simulink model "SPGF_FSK_0000_R2020b"  (R2020b)
settings: Solver=ode4  StartTime=0.0  StopTime=1.4  FixedStep=50e-6/50  RelTol=1e-3  EnableMultiTasking=on
undefined symbols (not defined in the file): D11, Delta
libraries: powerlib x2546, powerlib_meascontrol x183, simulink x24
(part 5 of 34)

== system SPGF_FSK_0000_R2020b/W15 ==
  DPL : Subsystem  Commented=on  mask{N=6, Frequency=[50], R_matrix=[0.615576503610254 0.0494305423965082 0.0494304372287521 0.0494304372287521 0.0494304372287521 0.0494304372287521;0.0494305423965082 0.673800204514058 0.0494304372287521 0.0494304372287521 0.0494304372287521 0.0494304372287521;0.0494304372287521 0.0494304372287521 0.615577059271979 0.0494310980582332 0.0494309929448645 0.0494309929448645;0.0494304372287521 0.0494304372287521 0.0494310980582332 0.673800760175783 0.0494309929448645 0.0494309929448645;0.0494304372287521 0.0494304372287521 0.0494309929448645 0.0494309929448645 0.615577059271979 0.0494310980582332;0.0494304372287521 0.0494304372287521 0.0494309929448645 0.0494309929448645 0.0494310980582332 0.673800760175783], L_matrix=[0.00267974020684065 0.00245992521794015 0.00224611545694793 0.00224611545694793 0.00224611545694793 0.00224611545694793;0.00245992521794015 0.00245824456959281 0.00224611545694793 0.00224611545694793 0.00224611545694793 0.00224611545694793;0.00224611545694793 0.00224611545694793 0.00260525290490007 0.00238543791599956 0.00226842802338409 0.00226842802338409;0.00224611545694793 0.00224611545694793 0.00238543791599956 0.00238375726765222 0.00226842802338409 0.00226842802338409;0.00224611545694793 0.00224611545694793 0.00226842802338409 0.00226842802338409 0.00260525290490007 0.00238543791599956;0.00224611545694793 0.00224611545694793 0.00226842802338409 0.00226842802338409 0.00238543791599956 0.00238375726765222], C_matrix=[1.52007862009692e-07 -1.52007862009692e-07 0 0 0 0;-1.52007862009692e-07 3.21528164058002e-07 0 0 0 0;0 0 1.52007862009692e-07 -1.52007862009692e-07 0 0;0 0 -1.52007862009692e-07 3.21528164058002e-07 0 0;0 0 0 0 1.52007862009692e-07 -1.52007862009692e-07;0 0 0 0 -1.52007862009692e-07 3.21528164058002e-07], Rg_matrix=[1047017.83833883 -1047017.83833883 Inf Inf Inf -Inf;-1047017.83833883 494995.340635804 Inf Inf Inf -Inf;Inf Inf 1047017.83833883 -1047017.83833883 Inf -Inf;Inf Inf -1047017.83833883 494995.340635804 Inf -Inf;Inf Inf Inf Inf 1047017.83833883 -1047017.83833883;Inf Inf Inf Inf -1047017.83833883 494995.340635804], LineLength=[0.5]}
      mask prompts: N "Number of phases [N]"; Frequency "Frequency used for rlc specification [Hz]:"; R_matrix "Resistance per unit length [Ohms/km] NxN matrix"; L_matrix "Inductance per unit length [H/km] NxN matrix"; C_matrix "Capacitance per unit length [F/km] NxN matrix"; Rg_matrix "Resistance shunt matrix 6*6 [Ohm*km]"; LineLength "Line Length(km)"
      mask init:
      | % Rloss=1/(2*pi*Frequency*C_matrix(1,1)*TangLoss);
      | Rg_matrix=Rg_matrix./LineLength;
      mask Display:
      | port_label('lconn',1,'A');
      | port_label('lconn',2,'B');
      | port_label('lconn',3,'C');
      | 
      | port_label('rconn',1,'a');
      | port_label('rconn',2,'b');
      | port_label('rconn',3,'c');
      | 
      | disp('1x50');
  Pi : Subsystem  mask{R0=0.589, X0=0.09, Cp0=0.29, tg=2, Frequency=[50], LineLength=[0.5]}
      mask prompts: R0 "Удельное активное сопротивление, Ом/км"; X0 "Удельное индуктивное сопротивление, Ом/км"; Cp0 "Удельная рабочая емкость, мкФ/км"; tg "Тангенс диэлектрических потерь, %"; Frequency "Частота сети, Гц"; LineLength "Длина линии, км"
      mask init:
      | R=R0*LineLength;
      | L=X0*LineLength/(2*pi*Frequency);
      | Cp=Cp0*LineLength*1e-6;
      | Cmf=0.1525*Cp;
      | Cfg=0.56*Cp;
      | tg_pu=tg/100;
      | 
      | Rmf=1/(Cmf*2*pi*Frequency*tg_pu);
      | Rfg=1/(Cfg*2*pi*Frequency*tg_pu);
      mask Display:
      | port_label('lconn',1,'A');
      | port_label('lconn',2,'B');
      | port_label('lconn',3,'C');
      | 
      | port_label('rconn',1,'a');
      | port_label('rconn',2,'b');
      | port_label('rconn',3,'c');
      | 
      | disp('1x50');
  Q : Subsystem
  concentrated : Subsystem  Commented=on  mask{N=6, Frequency=[50], R_matrix=[0.615576503610254 0.0494305423965082 0.0494304372287521 0.0494304372287521 0.0494304372287521 0.0494304372287521;0.0494305423965082 0.673800204514058 0.0494304372287521 0.0494304372287521 0.0494304372287521 0.0494304372287521;0.0494304372287521 0.0494304372287521 0.615577059271979 0.0494310980582332 0.0494309929448645 0.0494309929448645;0.0494304372287521 0.0494304372287521 0.0494310980582332 0.673800760175783 0.0494309929448645 0.0494309929448645;0.0494304372287521 0.0494304372287521 0.0494309929448645 0.0494309929448645 0.615577059271979 0.0494310980582332;0.0494304372287521 0.0494304372287521 0.0494309929448645 0.0494309929448645 0.0494310980582332 0.673800760175783], L_matrix=[0.00267974020684065 0.00245992521794015 0.00224611545694793 0.00224611545694793 0.00224611545694793 0.00224611545694793;0.00245992521794015 0.00245824456959281 0.00224611545694793 0.00224611545694793 0.00224611545694793 0.00224611545694793;0.00224611545694793 0.00224611545694793 0.00260525290490007 0.00238543791599956 0.00226842802338409 0.00226842802338409;0.00224611545694793 0.00224611545694793 0.00238543791599956 0.00238375726765222 0.00226842802338409 0.00226842802338409;0.00224611545694793 0.00224611545694793 0.00226842802338409 0.00226842802338409 0.00260525290490007 0.00238543791599956;0.00224611545694793 0.00224611545694793 0.00226842802338409 0.00226842802338409 0.00238543791599956 0.00238375726765222], C_matrix=[1.52007862009692e-07 -1.52007862009692e-07 0 0 0 0;-1.52007862009692e-07 3.21528164058002e-07 0 0 0 0;0 0 1.52007862009692e-07 -1.52007862009692e-07 0 0;0 0 -1.52007862009692e-07 3.21528164058002e-07 0 0;0 0 0 0 1.52007862009692e-07 -1.52007862009692e-07;0 0 0 0 -1.52007862009692e-07 3.21528164058002e-07], Rg_matrix=[1047017.83833883 -1047017.83833883 Inf Inf Inf -Inf;-1047017.83833883 494995.340635804 Inf Inf Inf -Inf;Inf Inf 1047017.83833883 -1047017.83833883 Inf -Inf;Inf Inf -1047017.83833883 494995.340635804 Inf -Inf;Inf Inf Inf Inf 1047017.83833883 -1047017.83833883;Inf Inf Inf Inf -1047017.83833883 494995.340635804], LineLength=[0.5]}
      mask prompts: N "Number of phases [N]"; Frequency "Frequency [Hz]:"; R_matrix "Resistance matrix 6*6 [Ohm/km]"; L_matrix "Inductance matrix 6*6 [H/km]"; C_matrix "Capacitance matrix 6*6 [F/km]"; Rg_matrix "Resistance shunt matrix 6*6 [Ohm*km]"; LineLength "Line Length(km)"
      mask init: same as SPGF_FSK_0000_R2020b/W11/concentrated
      mask Display:
      | port_label('lconn',1,'A');
      | port_label('lconn',2,'B');
      | port_label('lconn',3,'C');
      | 
      | port_label('rconn',1,'a');
      | port_label('rconn',2,'b');
      | port_label('rconn',3,'c');
      | 
      | disp('1x50');
  a : PMIOPort  Side=Right
  b : PMIOPort  Port=2  Side=Right
  c : PMIOPort  Port=3  Side=Right
  A : PMIOPort  Port=4  Side=Left
  B : PMIOPort  Port=5  Side=Left
  C : PMIOPort  Port=6  Side=Left
  connections:
  B/RConn1 -- Pi/LConn2 -- DPL/LConn2 -- concentrated/LConn2
  Pi/RConn3 -- Q/LConn3 -- DPL/RConn3 -- concentrated/RConn3
  Pi/RConn1 -- Q/LConn1 -- DPL/RConn1 -- concentrated/RConn1
  Pi/RConn2 -- Q/LConn2 -- DPL/RConn2 -- concentrated/RConn2
  C/RConn1 -- Pi/LConn3 -- concentrated/LConn3 -- DPL/LConn3
  A/RConn1 -- Pi/LConn1 -- DPL/LConn1 -- concentrated/LConn1
  Q/RConn2 -- b/RConn1
  Q/RConn3 -- c/RConn1
  Q/RConn1 -- a/RConn1

== system SPGF_FSK_0000_R2020b/W21 ==
  DPL : Subsystem  Commented=on  mask{N=6, Frequency=[50], R_matrix=[0.238533070672438 0.0494305686816904 0.0494306099166724 0.0494306099166724 0.0494306099166724 0.0494306099166724;0.0494305686816904 0.477102342029173 0.0494306099166724 0.0494306099166724 0.0494306099166724 0.0494306099166724;0.0494306099166724 0.0494306099166724 0.238533799046727 0.0494312970559801 0.0494313383808651 0.0494313383808651;0.0494306099166724 0.0494306099166724 0.0494312970559801 0.477103070403462 0.0494313383808651 0.0494313383808651;0.0494306099166724 0.0494306099166724 0.0494313383808651 0.0494313383808651 0.238533799046727 0.0494312970559801;0.0494306099166724 0.0494306099166724 0.0494313383808651 0.0494313383808651 0.0494312970559801 0.477103070403462], L_matrix=[0.00256327039444001 0.00239846064177441 0.00219197508429097 0.00219197508429097 0.00219197508429097 0.00219197508429097;0.00239846064177441 0.00239704374511945 0.00219197508429097 0.00219197508429097 0.00219197508429097 0.00219197508429097;0.00219197508429097 0.00219197508429097 0.00248961125686914 0.00232480150420353 0.00221428709466139 0.00221428709466139;0.00219197508429097 0.00219197508429097 0.00232480150420353 0.00232338460754857 0.00221428709466139 0.00221428709466139;0.00219197508429097 0.00219197508429097 0.00221428709466139 0.00221428709466139 0.00248961125686914 0.00232480150420353;0.00219197508429097 0.00219197508429097 0.00221428709466139 0.00221428709466139 0.00232480150420353 0.00232338460754857], C_matrix=[2.26444096304697e-07 -2.26444096304697e-07 0 0 0 0;-2.26444096304697e-07 4.01872387610564e-07 0 0 0 0;0 0 2.26444096304697e-07 -2.26444096304697e-07 0 0;0 0 -2.26444096304697e-07 4.01872387610564e-07 0 0;0 0 0 0 2.26444096304697e-07 -2.26444096304697e-07;0 0 0 0 -2.26444096304697e-07 4.01872387610564e-07], Rg_matrix=[702844.303247989 -702844.303247989 Inf Inf Inf -Inf;-702844.303247989 396033.537009577 Inf Inf Inf -Inf;Inf Inf 702844.303247989 -702844.303247989 Inf -Inf;Inf Inf -702844.303247989 396033.537009577 Inf -Inf;Inf Inf Inf Inf 702844.303247989 -702844.303247989;Inf Inf Inf Inf -702844.303247989 396033.537009577], LineLength=[0.8]}
      mask prompts: N "Number of phases [N]"; Frequency "Frequency used for rlc specification [Hz]:"; R_matrix "Resistance per unit length [Ohms/km] NxN matrix"; L_matrix "Inductance per unit length [H/km] NxN matrix"; C_matrix "Capacitance per unit length [F/km] NxN matrix"; Rg_matrix "Resistance shunt matrix 6*6 [Ohm*km]"; LineLength "Line Length(km)"
      mask init:
      | % Rloss=1/(2*pi*Frequency*C_matrix(1,1)*TangLoss);
      | Rg_matrix=Rg_matrix./LineLength;
      mask Display:
      | port_label('lconn',1,'A');
      | port_label('lconn',2,'B');
      | port_label('lconn',3,'C');
      | 
      | port_label('rconn',1,'a');
      | port_label('rconn',2,'b');
      | port_label('rconn',3,'c');
      | 
      | disp('1x150');
  Pi : Subsystem  mask{R0=0.196, X0=0.079, Cp0=0.44, tg=2, Frequency=[50], LineLength=[0.8]}
      mask prompts: R0 "Удельное активное сопротивление, Ом/км"; X0 "Удельное индуктивное сопротивление, Ом/км"; Cp0 "Удельная рабочая емкость, мкФ/км"; tg "Тангенс диэлектрических потерь, %"; Frequency "Частота сети, Гц"; LineLength "Длина линии, км"
      mask init:
      | R=R0*LineLength;
      | L=X0*LineLength/(2*pi*Frequency);
      | Cp=Cp0*LineLength*1e-6;
      | Cmf=0.1525*Cp;
      | Cfg=0.56*Cp;
      | tg_pu=tg/100;
      | 
      | Rmf=1/(Cmf*2*pi*Frequency*tg_pu);
      | Rfg=1/(Cfg*2*pi*Frequency*tg_pu);
      mask Display:
      | port_label('lconn',1,'A');
      | port_label('lconn',2,'B');
      | port_label('lconn',3,'C');
      | 
      | port_label('rconn',1,'a');
      | port_label('rconn',2,'b');
      | port_label('rconn',3,'c');
      | 
      | disp('1x150');
  Q : Subsystem
  concentrated : Subsystem  Commented=on  mask{N=6, Frequency=[50], R_matrix=[0.238533070672438 0.0494305686816904 0.0494306099166724 0.0494306099166724 0.0494306099166724 0.0494306099166724;0.0494305686816904 0.477102342029173 0.0494306099166724 0.0494306099166724 0.0494306099166724 0.0494306099166724;0.0494306099166724 0.0494306099166724 0.238533799046727 0.0494312970559801 0.0494313383808651 0.0494313383808651;0.0494306099166724 0.0494306099166724 0.0494312970559801 0.477103070403462 0.0494313383808651 0.0494313383808651;0.0494306099166724 0.0494306099166724 0.0494313383808651 0.0494313383808651 0.238533799046727 0.0494312970559801;0.0494306099166724 0.0494306099166724 0.0494313383808651 0.0494313383808651 0.0494312970559801 0.477103070403462], L_matrix=[0.00256327039444001 0.00239846064177441 0.00219197508429097 0.00219197508429097 0.00219197508429097 0.00219197508429097;0.00239846064177441 0.00239704374511945 0.00219197508429097 0.00219197508429097 0.00219197508429097 0.00219197508429097;0.00219197508429097 0.00219197508429097 0.00248961125686914 0.00232480150420353 0.00221428709466139 0.00221428709466139;0.00219197508429097 0.00219197508429097 0.00232480150420353 0.00232338460754857 0.00221428709466139 0.00221428709466139;0.00219197508429097 0.00219197508429097 0.00221428709466139 0.00221428709466139 0.00248961125686914 0.00232480150420353;0.00219197508429097 0.00219197508429097 0.00221428709466139 0.00221428709466139 0.00232480150420353 0.00232338460754857], C_matrix=[2.26444096304697e-07 -2.26444096304697e-07 0 0 0 0;-2.26444096304697e-07 4.01872387610564e-07 0 0 0 0;0 0 2.26444096304697e-07 -2.26444096304697e-07 0 0;0 0 -2.26444096304697e-07 4.01872387610564e-07 0 0;0 0 0 0 2.26444096304697e-07 -2.26444096304697e-07;0 0 0 0 -2.26444096304697e-07 4.01872387610564e-07], Rg_matrix=[702844.303247989 -702844.303247989 Inf Inf Inf -Inf;-702844.303247989 396033.537009577 Inf Inf Inf -Inf;Inf Inf 702844.303247989 -702844.303247989 Inf -Inf;Inf Inf -702844.303247989 396033.537009577 Inf -Inf;Inf Inf Inf Inf 702844.303247989 -702844.303247989;Inf Inf Inf Inf -702844.303247989 396033.537009577], LineLength=[0.8]}
      mask prompts: N "Number of phases [N]"; Frequency "Frequency [Hz]:"; R_matrix "Resistance matrix 6*6 [Ohm/km]"; L_matrix "Inductance matrix 6*6 [H/km]"; C_matrix "Capacitance matrix 6*6 [F/km]"; Rg_matrix "Resistance shunt matrix 6*6 [Ohm*km]"; LineLength "Line Length(km)"
      mask init: same as SPGF_FSK_0000_R2020b/W11/concentrated
      mask Display:
      | port_label('lconn',1,'A');
      | port_label('lconn',2,'B');
      | port_label('lconn',3,'C');
      | 
      | port_label('rconn',1,'a');
      | port_label('rconn',2,'b');
      | port_label('rconn',3,'c');
      | 
      | disp('1x150');
  a : PMIOPort  Side=Right
  b : PMIOPort  Port=2  Side=Right
  c : PMIOPort  Port=3  Side=Right
  A : PMIOPort  Port=4  Side=Left
  B : PMIOPort  Port=5  Side=Left
  C : PMIOPort  Port=6  Side=Left
  connections:
  A/RConn1 -- Pi/LConn1 -- DPL/LConn1 -- concentrated/LConn1
  C/RConn1 -- Pi/LConn3 -- concentrated/LConn3 -- DPL/LConn3
  Pi/RConn2 -- Q/LConn2 -- DPL/RConn2 -- concentrated/RConn2
  Pi/RConn1 -- Q/LConn1 -- DPL/RConn1 -- concentrated/RConn1
  Pi/RConn3 -- Q/LConn3 -- DPL/RConn3 -- concentrated/RConn3
  B/RConn1 -- Pi/LConn2 -- DPL/LConn2 -- concentrated/LConn2
  Q/RConn3 -- c/RConn1
  Q/RConn2 -- b/RConn1
  Q/RConn1 -- a/RConn1

== system SPGF_FSK_0000_R2020b/W22 ==
  DPL : Subsystem  Commented=on  mask{N=6, Frequency=[50], R_matrix=[0.347601410823579 0.0494303286168989 0.0494305228057156 0.0494305228057156 0.0494305228057156 0.0494305228057156;0.0494303286168989 0.63357380919679 0.0494305228057156 0.0494305228057156 0.0494305228057156 0.0494305228057156;0.0494305228057156 0.0494305228057156 0.347602052073771 0.0494309698670905 0.0494311641268522 0.0494311641268522;0.0494305228057156 0.0494305228057156 0.0494309698670905 0.633574450446981 0.0494311641268522 0.0494311641268522;0.0494305228057156 0.0494305228057156 0.0494311641268522 0.0494311641268522 0.347602052073771 0.0494309698670905;0.0494305228057156 0.0494305228057156 0.0494311641268522 0.0494311641268522 0.0494309698670905 0.633574450446981], L_matrix=[0.00260859879857304 0.00242332383525137 0.00221745883616686 0.00221745883616686 0.00221745883616686 0.00221745883616686;0.00242332383525137 0.00242198857850016 0.00221745883616686 0.00221745883616686 0.00221745883616686 0.00221745883616686;0.00221745883616686 0.00221745883616686 0.00253519514382882 0.00234992018050715 0.00223977112704788 0.00223977112704788;0.00221745883616686 0.00221745883616686 0.00234992018050715 0.00234858492375594 0.00223977112704788 0.00223977112704788;0.00221745883616686 0.00221745883616686 0.00223977112704788 0.00223977112704788 0.00253519514382882 0.00234992018050715;0.00221745883616686 0.00221745883616686 0.00223977112704788 0.00223977112704788 0.00234992018050715 0.00234858492375594], C_matrix=[1.90757475136094e-07 -1.90757475136094e-07 0 0 0 0;-1.90757475136094e-07 3.66052807704686e-07 0 0 0 0;0 0 1.90757475136094e-07 -1.90757475136094e-07 0 0;0 0 -1.90757475136094e-07 3.66052807704686e-07 0 0;0 0 0 0 1.90757475136094e-07 -1.90757475136094e-07;0 0 0 0 -1.90757475136094e-07 3.66052807704686e-07], Rg_matrix=[834331.357019417 -834331.357019417 Inf Inf Inf -Inf;-834331.357019417 434786.838789375 Inf Inf Inf -Inf;Inf Inf 834331.357019417 -834331.357019417 Inf -Inf;Inf Inf -834331.357019417 434786.838789375 Inf -Inf;Inf Inf Inf Inf 834331.357019417 -834331.357019417;Inf Inf Inf Inf -834331.357019417 434786.838789375], LineLength=[0.3]}
      mask prompts: N "Number of phases [N]"; Frequency "Frequency used for rlc specification [Hz]:"; R_matrix "Resistance per unit length [Ohms/km] NxN matrix"; L_matrix "Inductance per unit length [H/km] NxN matrix"; C_matrix "Capacitance per unit length [F/km] NxN matrix"; Rg_matrix "Resistance shunt matrix 6*6 [Ohm*km]"; LineLength "Line Length(km)"
      mask init:
      | % Rloss=1/(2*pi*Frequency*C_matrix(1,1)*TangLoss);
      | Rg_matrix=Rg_matrix./LineLength;
      mask Display:
      | port_label('lconn',1,'A');
      | port_label('lconn',2,'B');
      | port_label('lconn',3,'C');
      | 
      | port_label('rconn',1,'a');
      | port_label('rconn',2,'b');
      | port_label('rconn',3,'c');
      | 
      | disp('1x95');
  Pi : Subsystem  mask{R0=0.31, X0=0.083, Cp0=0.35, tg=2, Frequency=[50], LineLength=[0.3]}
      mask prompts: R0 "Удельное активное сопротивление, Ом/км"; X0 "Удельное индуктивное сопротивление, Ом/км"; Cp0 "Удельная рабочая емкость, мкФ/км"; tg "Тангенс диэлектрических потерь, %"; Frequency "Частота сети, Гц"; LineLength "Длина линии, км"
      mask init:
      | R=R0*LineLength;
      | L=X0*LineLength/(2*pi*Frequency);
      | Cp=Cp0*LineLength*1e-6;
      | Cmf=0.1525*Cp;
      | Cfg=0.56*Cp;
      | tg_pu=tg/100;
      | 
      | Rmf=1/(Cmf*2*pi*Frequency*tg_pu);
      | Rfg=1/(Cfg*2*pi*Frequency*tg_pu);
      mask Display:
      | port_label('lconn',1,'A');
      | port_label('lconn',2,'B');
      | port_label('lconn',3,'C');
      | 
      | port_label('rconn',1,'a');
      | port_label('rconn',2,'b');
      | port_label('rconn',3,'c');
      | 
      | disp('1x95');
  Q : Subsystem
  concentrated : Subsystem  Commented=on  mask{N=6, Frequency=[50], R_matrix=[0.347601410823579 0.0494303286168989 0.0494305228057156 0.0494305228057156 0.0494305228057156 0.0494305228057156;0.0494303286168989 0.63357380919679 0.0494305228057156 0.0494305228057156 0.0494305228057156 0.0494305228057156;0.0494305228057156 0.0494305228057156 0.347602052073771 0.0494309698670905 0.0494311641268522 0.0494311641268522;0.0494305228057156 0.0494305228057156 0.0494309698670905 0.633574450446981 0.0494311641268522 0.0494311641268522;0.0494305228057156 0.0494305228057156 0.0494311641268522 0.0494311641268522 0.347602052073771 0.0494309698670905;0.0494305228057156 0.0494305228057156 0.0494311641268522 0.0494311641268522 0.0494309698670905 0.633574450446981], L_matrix=[0.00260859879857304 0.00242332383525137 0.00221745883616686 0.00221745883616686 0.00221745883616686 0.00221745883616686;0.00242332383525137 0.00242198857850016 0.00221745883616686 0.00221745883616686 0.00221745883616686 0.00221745883616686;0.00221745883616686 0.00221745883616686 0.00253519514382882 0.00234992018050715 0.00223977112704788 0.00223977112704788;0.00221745883616686 0.00221745883616686 0.00234992018050715 0.00234858492375594 0.00223977112704788 0.00223977112704788;0.00221745883616686 0.00221745883616686 0.00223977112704788 0.00223977112704788 0.00253519514382882 0.00234992018050715;0.00221745883616686 0.00221745883616686 0.00223977112704788 0.00223977112704788 0.00234992018050715 0.00234858492375594], C_matrix=[1.90757475136094e-07 -1.90757475136094e-07 0 0 0 0;-1.90757475136094e-07 3.66052807704686e-07 0 0 0 0;0 0 1.90757475136094e-07 -1.90757475136094e-07 0 0;0 0 -1.90757475136094e-07 3.66052807704686e-07 0 0;0 0 0 0 1.90757475136094e-07 -1.90757475136094e-07;0 0 0 0 -1.90757475136094e-07 3.66052807704686e-07], Rg_matrix=[834331.357019417 -834331.357019417 Inf Inf Inf -Inf;-834331.357019417 434786.838789375 Inf Inf Inf -Inf;Inf Inf 834331.357019417 -834331.357019417 Inf -Inf;Inf Inf -834331.357019417 434786.838789375 Inf -Inf;Inf Inf Inf Inf 834331.357019417 -834331.357019417;Inf Inf Inf Inf -834331.357019417 434786.838789375], LineLength=[0.3]}
      mask prompts: N "Number of phases [N]"; Frequency "Frequency [Hz]:"; R_matrix "Resistance matrix 6*6 [Ohm/km]"; L_matrix "Inductance matrix 6*6 [H/km]"; C_matrix "Capacitance matrix 6*6 [F/km]"; Rg_matrix "Resistance shunt matrix 6*6 [Ohm*km]"; LineLength "Line Length(km)"
      mask init: same as SPGF_FSK_0000_R2020b/W11/concentrated
      mask Display:
      | port_label('lconn',1,'A');
      | port_label('lconn',2,'B');
      | port_label('lconn',3,'C');
      | 
      | port_label('rconn',1,'a');
      | port_label('rconn',2,'b');
      | port_label('rconn',3,'c');
      | 
      | disp('1x95');
  a : PMIOPort  Side=Right
  b : PMIOPort  Port=2  Side=Right
  c : PMIOPort  Port=3  Side=Right
  A : PMIOPort  Port=4  Side=Left
  B : PMIOPort  Port=5  Side=Left
  C : PMIOPort  Port=6  Side=Left
  connections:
  A/RConn1 -- concentrated/LConn1 -- DPL/LConn1 -- Pi/LConn1
  C/RConn1 -- DPL/LConn3 -- concentrated/LConn3 -- Pi/LConn3
  concentrated/RConn2 -- Q/LConn2 -- DPL/RConn2 -- Pi/RConn2
  concentrated/RConn1 -- Q/LConn1 -- DPL/RConn1 -- Pi/RConn1
  concentrated/RConn3 -- Q/LConn3 -- DPL/RConn3 -- Pi/RConn3
  B/RConn1 -- concentrated/LConn2 -- DPL/LConn2 -- Pi/LConn2
  Q/RConn2 -- b/RConn1
  Q/RConn1 -- a/RConn1
  Q/RConn3 -- c/RConn1

== system SPGF_FSK_0000_R2020b/W31 ==
  DPL : Subsystem  Commented=on  mask{N=6, Frequency=[50], R_matrix=[0.238533070672438 0.0494305686816904 0.0494306099166724 0.0494306099166724 0.0494306099166724 0.0494306099166724;0.0494305686816904 0.477102342029173 0.0494306099166724 0.0494306099166724 0.0494306099166724 0.0494306099166724;0.0494306099166724 0.0494306099166724 0.238533799046727 0.0494312970559801 0.0494313383808651 0.0494313383808651;0.0494306099166724 0.0494306099166724 0.0494312970559801 0.477103070403462 0.0494313383808651 0.0494313383808651;0.0494306099166724 0.0494306099166724 0.0494313383808651 0.0494313383808651 0.238533799046727 0.0494312970559801;0.0494306099166724 0.0494306099166724 0.0494313383808651 0.0494313383808651 0.0494312970559801 0.477103070403462], L_matrix=[0.00256327039444001 0.00239846064177441 0.00219197508429097 0.00219197508429097 0.00219197508429097 0.00219197508429097;0.00239846064177441 0.00239704374511945 0.00219197508429097 0.00219197508429097 0.00219197508429097 0.00219197508429097;0.00219197508429097 0.00219197508429097 0.00248961125686914 0.00232480150420353 0.00221428709466139 0.00221428709466139;0.00219197508429097 0.00219197508429097 0.00232480150420353 0.00232338460754857 0.00221428709466139 0.00221428709466139;0.00219197508429097 0.00219197508429097 0.00221428709466139 0.00221428709466139 0.00248961125686914 0.00232480150420353;0.00219197508429097 0.00219197508429097 0.00221428709466139 0.00221428709466139 0.00232480150420353 0.00232338460754857], C_matrix=[2.26444096304697e-07 -2.26444096304697e-07 0 0 0 0;-2.26444096304697e-07 4.01872387610564e-07 0 0 0 0;0 0 2.26444096304697e-07 -2.26444096304697e-07 0 0;0 0 -2.26444096304697e-07 4.01872387610564e-07 0 0;0 0 0 0 2.26444096304697e-07 -2.26444096304697e-07;0 0 0 0 -2.26444096304697e-07 4.01872387610564e-07], Rg_matrix=[702844.303247989 -702844.303247989 Inf Inf Inf -Inf;-702844.303247989 396033.537009577 Inf Inf Inf -Inf;Inf Inf 702844.303247989 -702844.303247989 Inf -Inf;Inf Inf -702844.303247989 396033.537009577 Inf -Inf;Inf Inf Inf Inf 702844.303247989 -702844.303247989;Inf Inf Inf Inf -702844.303247989 396033.537009577], LineLength=[0.9]}
      mask prompts: N "Number of phases [N]"; Frequency "Frequency used for rlc specification [Hz]:"; R_matrix "Resistance per unit length [Ohms/km] NxN matrix"; L_matrix "Inductance per unit length [H/km] NxN matrix"; C_matrix "Capacitance per unit length [F/km] NxN matrix"; Rg_matrix "Resistance shunt matrix 6*6 [Ohm*km]"; LineLength "Line Length(km)"
      mask init:
      | % Rloss=1/(2*pi*Frequency*C_matrix(1,1)*TangLoss);
      | Rg_matrix=Rg_matrix./LineLength;
      mask Display:
      | port_label('lconn',1,'A');
      | port_label('lconn',2,'B');
      | port_label('lconn',3,'C');
      | 
      | port_label('rconn',1,'a');
      | port_label('rconn',2,'b');
      | port_label('rconn',3,'c');
      | 
      | disp('1x150');
  Pi : Subsystem  mask{R0=0.196, X0=0.079, Cp0=0.44, tg=2, Frequency=[50], LineLength=[0.9]}
      mask prompts: R0 "Удельное активное сопротивление, Ом/км"; X0 "Удельное индуктивное сопротивление, Ом/км"; Cp0 "Удельная рабочая емкость, мкФ/км"; tg "Тангенс диэлектрических потерь, %"; Frequency "Частота сети, Гц"; LineLength "Длина линии, км"
      mask init:
      | R=R0*LineLength;
      | L=X0*LineLength/(2*pi*Frequency);
      | Cp=Cp0*LineLength*1e-6;
      | Cmf=0.1525*Cp;
      | Cfg=0.56*Cp;
      | tg_pu=tg/100;
      | 
      | Rmf=1/(Cmf*2*pi*Frequency*tg_pu);
      | Rfg=1/(Cfg*2*pi*Frequency*tg_pu);
      mask Display:
      | port_label('lconn',1,'A');
      | port_label('lconn',2,'B');
      | port_label('lconn',3,'C');
      | 
      | port_label('rconn',1,'a');
      | port_label('rconn',2,'b');
      | port_label('rconn',3,'c');
      | 
      | disp('1x150');
  Q : Subsystem
  concentrated : Subsystem  Commented=on  mask{N=6, Frequency=[50], R_matrix=[0.238533070672438 0.0494305686816904 0.0494306099166724 0.0494306099166724 0.0494306099166724 0.0494306099166724;0.0494305686816904 0.477102342029173 0.0494306099166724 0.0494306099166724 0.0494306099166724 0.0494306099166724;0.0494306099166724 0.0494306099166724 0.238533799046727 0.0494312970559801 0.0494313383808651 0.0494313383808651;0.0494306099166724 0.0494306099166724 0.0494312970559801 0.477103070403462 0.0494313383808651 0.0494313383808651;0.0494306099166724 0.0494306099166724 0.0494313383808651 0.0494313383808651 0.238533799046727 0.0494312970559801;0.0494306099166724 0.0494306099166724 0.0494313383808651 0.0494313383808651 0.0494312970559801 0.477103070403462], L_matrix=[0.00256327039444001 0.00239846064177441 0.00219197508429097 0.00219197508429097 0.00219197508429097 0.00219197508429097;0.00239846064177441 0.00239704374511945 0.00219197508429097 0.00219197508429097 0.00219197508429097 0.00219197508429097;0.00219197508429097 0.00219197508429097 0.00248961125686914 0.00232480150420353 0.00221428709466139 0.00221428709466139;0.00219197508429097 0.00219197508429097 0.00232480150420353 0.00232338460754857 0.00221428709466139 0.00221428709466139;0.00219197508429097 0.00219197508429097 0.00221428709466139 0.00221428709466139 0.00248961125686914 0.00232480150420353;0.00219197508429097 0.00219197508429097 0.00221428709466139 0.00221428709466139 0.00232480150420353 0.00232338460754857], C_matrix=[2.26444096304697e-07 -2.26444096304697e-07 0 0 0 0;-2.26444096304697e-07 4.01872387610564e-07 0 0 0 0;0 0 2.26444096304697e-07 -2.26444096304697e-07 0 0;0 0 -2.26444096304697e-07 4.01872387610564e-07 0 0;0 0 0 0 2.26444096304697e-07 -2.26444096304697e-07;0 0 0 0 -2.26444096304697e-07 4.01872387610564e-07], Rg_matrix=[702844.303247989 -702844.303247989 Inf Inf Inf -Inf;-702844.303247989 396033.537009577 Inf Inf Inf -Inf;Inf Inf 702844.303247989 -702844.303247989 Inf -Inf;Inf Inf -702844.303247989 396033.537009577 Inf -Inf;Inf Inf Inf Inf 702844.303247989 -702844.303247989;Inf Inf Inf Inf -702844.303247989 396033.537009577], LineLength=[0.9]}
      mask prompts: N "Number of phases [N]"; Frequency "Frequency [Hz]:"; R_matrix "Resistance matrix 6*6 [Ohm/km]"; L_matrix "Inductance matrix 6*6 [H/km]"; C_matrix "Capacitance matrix 6*6 [F/km]"; Rg_matrix "Resistance shunt matrix 6*6 [Ohm*km]"; LineLength "Line Length(km)"
      mask init: same as SPGF_FSK_0000_R2020b/W11/concentrated
      mask Display:
      | port_label('lconn',1,'A');
      | port_label('lconn',2,'B');
      | port_label('lconn',3,'C');
      | 
      | port_label('rconn',1,'a');
      | port_label('rconn',2,'b');
      | port_label('rconn',3,'c');
      | 
      | disp('1x150');
  a : PMIOPort  Side=Right
  b : PMIOPort  Port=2  Side=Right
  c : PMIOPort  Port=3  Side=Right
  A : PMIOPort  Port=4  Side=Left
  B : PMIOPort  Port=5  Side=Left
  C : PMIOPort  Port=6  Side=Left
  connections:
  Q/RConn1 -- a/RConn1
  Q/RConn2 -- b/RConn1
  Q/RConn3 -- c/RConn1
  Pi/LConn2 -- concentrated/LConn2 -- DPL/LConn2 -- B/RConn1
  Pi/RConn3 -- Q/LConn3 -- concentrated/RConn3 -- DPL/RConn3
  Pi/RConn1 -- Q/LConn1 -- concentrated/RConn1 -- DPL/RConn1
  Pi/RConn2 -- Q/LConn2 -- concentrated/RConn2 -- DPL/RConn2
  Pi/LConn3 -- concentrated/LConn3 -- DPL/LConn3 -- C/RConn1
  Pi/LConn1 -- concentrated/LConn1 -- DPL/LConn1 -- A/RConn1

== system SPGF_FSK_0000_R2020b/W32 ==
  DPL : Subsystem  Commented=on  mask{N=6, Frequency=[50], R_matrix=[0.347601410823579 0.0494303286168989 0.0494305228057156 0.0494305228057156 0.0494305228057156 0.0494305228057156;0.0494303286168989 0.63357380919679 0.0494305228057156 0.0494305228057156 0.0494305228057156 0.0494305228057156;0.0494305228057156 0.0494305228057156 0.347602052073771 0.0494309698670905 0.0494311641268522 0.0494311641268522;0.0494305228057156 0.0494305228057156 0.0494309698670905 0.633574450446981 0.0494311641268522 0.0494311641268522;0.0494305228057156 0.0494305228057156 0.0494311641268522 0.0494311641268522 0.347602052073771 0.0494309698670905;0.0494305228057156 0.0494305228057156 0.0494311641268522 0.0494311641268522 0.0494309698670905 0.633574450446981], L_matrix=[0.00260859879857304 0.00242332383525137 0.00221745883616686 0.00221745883616686 0.00221745883616686 0.00221745883616686;0.00242332383525137 0.00242198857850016 0.00221745883616686 0.00221745883616686 0.00221745883616686 0.00221745883616686;0.00221745883616686 0.00221745883616686 0.00253519514382882 0.00234992018050715 0.00223977112704788 0.00223977112704788;0.00221745883616686 0.00221745883616686 0.00234992018050715 0.00234858492375594 0.00223977112704788 0.00223977112704788;0.00221745883616686 0.00221745883616686 0.00223977112704788 0.00223977112704788 0.00253519514382882 0.00234992018050715;0.00221745883616686 0.00221745883616686 0.00223977112704788 0.00223977112704788 0.00234992018050715 0.00234858492375594], C_matrix=[1.90757475136094e-07 -1.90757475136094e-07 0 0 0 0;-1.90757475136094e-07 3.66052807704686e-07 0 0 0 0;0 0 1.90757475136094e-07 -1.90757475136094e-07 0 0;0 0 -1.90757475136094e-07 3.66052807704686e-07 0 0;0 0 0 0 1.90757475136094e-07 -1.90757475136094e-07;0 0 0 0 -1.90757475136094e-07 3.66052807704686e-07], Rg_matrix=[834331.357019417 -834331.357019417 Inf Inf Inf -Inf;-834331.357019417 434786.838789375 Inf Inf Inf -Inf;Inf Inf 834331.357019417 -834331.357019417 Inf -Inf;Inf Inf -834331.357019417 434786.838789375 Inf -Inf;Inf Inf Inf Inf 834331.357019417 -834331.357019417;Inf Inf Inf Inf -834331.357019417 434786.838789375], LineLength=[0.6]}
      mask prompts: N "Number of phases [N]"; Frequency "Frequency used for rlc specification [Hz]:"; R_matrix "Resistance per unit length [Ohms/km] NxN matrix"; L_matrix "Inductance per unit length [H/km] NxN matrix"; C_matrix "Capacitance per unit length [F/km] NxN matrix"; Rg_matrix "Resistance shunt matrix 6*6 [Ohm*km]"; LineLength "Line Length(km)"
      mask init:
      | % Rloss=1/(2*pi*Frequency*C_matrix(1,1)*TangLoss);
      | Rg_matrix=Rg_matrix./LineLength;
      mask Display:
      | port_label('lconn',1,'A');
      | port_label('lconn',2,'B');
      | port_label('lconn',3,'C');
      | 
      | port_label('rconn',1,'a');
      | port_label('rconn',2,'b');
      | port_label('rconn',3,'c');
      | 
      | disp('1x95');
  Pi : Subsystem  mask{R0=0.31, X0=0.083, Cp0=0.35, tg=2, Frequency=[50], LineLength=[0.6]}
      mask prompts: R0 "Удельное активное сопротивление, Ом/км"; X0 "Удельное индуктивное сопротивление, Ом/км"; Cp0 "Удельная рабочая емкость, мкФ/км"; tg "Тангенс диэлектрических потерь, %"; Frequency "Частота сети, Гц"; LineLength "Длина линии, км"
      mask init:
      | R=R0*LineLength;
      | L=X0*LineLength/(2*pi*Frequency);
      | Cp=Cp0*LineLength*1e-6;
      | Cmf=0.1525*Cp;
      | Cfg=0.56*Cp;
      | tg_pu=tg/100;
      | 
      | Rmf=1/(Cmf*2*pi*Frequency*tg_pu);
      | Rfg=1/(Cfg*2*pi*Frequency*tg_pu);
      mask Display:
      | port_label('lconn',1,'A');
      | port_label('lconn',2,'B');
      | port_label('lconn',3,'C');
      | 
      | port_label('rconn',1,'a');
      | port_label('rconn',2,'b');
      | port_label('rconn',3,'c');
      | 
      | disp('1x95');
  Q : Subsystem
  concentrated : Subsystem  Commented=on  mask{N=6, Frequency=[50], R_matrix=[0.347601410823579 0.0494303286168989 0.0494305228057156 0.0494305228057156 0.0494305228057156 0.0494305228057156;0.0494303286168989 0.63357380919679 0.0494305228057156 0.0494305228057156 0.0494305228057156 0.0494305228057156;0.0494305228057156 0.0494305228057156 0.347602052073771 0.0494309698670905 0.0494311641268522 0.0494311641268522;0.0494305228057156 0.0494305228057156 0.0494309698670905 0.633574450446981 0.0494311641268522 0.0494311641268522;0.0494305228057156 0.0494305228057156 0.0494311641268522 0.0494311641268522 0.347602052073771 0.0494309698670905;0.0494305228057156 0.0494305228057156 0.0494311641268522 0.0494311641268522 0.0494309698670905 0.633574450446981], L_matrix=[0.00260859879857304 0.00242332383525137 0.00221745883616686 0.00221745883616686 0.00221745883616686 0.00221745883616686;0.00242332383525137 0.00242198857850016 0.00221745883616686 0.00221745883616686 0.00221745883616686 0.00221745883616686;0.00221745883616686 0.00221745883616686 0.00253519514382882 0.00234992018050715 0.00223977112704788 0.00223977112704788;0.00221745883616686 0.00221745883616686 0.00234992018050715 0.00234858492375594 0.00223977112704788 0.00223977112704788;0.00221745883616686 0.00221745883616686 0.00223977112704788 0.00223977112704788 0.00253519514382882 0.00234992018050715;0.00221745883616686 0.00221745883616686 0.00223977112704788 0.00223977112704788 0.00234992018050715 0.00234858492375594], C_matrix=[1.90757475136094e-07 -1.90757475136094e-07 0 0 0 0;-1.90757475136094e-07 3.66052807704686e-07 0 0 0 0;0 0 1.90757475136094e-07 -1.90757475136094e-07 0 0;0 0 -1.90757475136094e-07 3.66052807704686e-07 0 0;0 0 0 0 1.90757475136094e-07 -1.90757475136094e-07;0 0 0 0 -1.90757475136094e-07 3.66052807704686e-07], Rg_matrix=[834331.357019417 -834331.357019417 Inf Inf Inf -Inf;-834331.357019417 434786.838789375 Inf Inf Inf -Inf;Inf Inf 834331.357019417 -834331.357019417 Inf -Inf;Inf Inf -834331.357019417 434786.838789375 Inf -Inf;Inf Inf Inf Inf 834331.357019417 -834331.357019417;Inf Inf Inf Inf -834331.357019417 434786.838789375], LineLength=[0.6]}
      mask prompts: N "Number of phases [N]"; Frequency "Frequency [Hz]:"; R_matrix "Resistance matrix 6*6 [Ohm/km]"; L_matrix "Inductance matrix 6*6 [H/km]"; C_matrix "Capacitance matrix 6*6 [F/km]"; Rg_matrix "Resistance shunt matrix 6*6 [Ohm*km]"; LineLength "Line Length(km)"
      mask init: same as SPGF_FSK_0000_R2020b/W11/concentrated
      mask Display:
      | port_label('lconn',1,'A');
      | port_label('lconn',2,'B');
      | port_label('lconn',3,'C');
      | 
      | port_label('rconn',1,'a');
      | port_label('rconn',2,'b');
      | port_label('rconn',3,'c');
      | 
      | disp('1x95');
  a : PMIOPort  Side=Right
  b : PMIOPort  Port=2  Side=Right
  c : PMIOPort  Port=3  Side=Right
  A : PMIOPort  Port=4  Side=Left
  B : PMIOPort  Port=5  Side=Left
  C : PMIOPort  Port=6  Side=Left
  connections:
  Q/RConn3 -- c/RConn1
  Q/RConn1 -- a/RConn1
  Q/RConn2 -- b/RConn1
  Pi/LConn2 -- DPL/LConn2 -- concentrated/LConn2 -- B/RConn1
  Pi/RConn3 -- Q/LConn3 -- DPL/RConn3 -- concentrated/RConn3
  Pi/RConn1 -- Q/LConn1 -- DPL/RConn1 -- concentrated/RConn1
  Pi/RConn2 -- Q/LConn2 -- DPL/RConn2 -- concentrated/RConn2
  Pi/LConn3 -- concentrated/LConn3 -- DPL/LConn3 -- C/RConn1
  Pi/LConn1 -- DPL/LConn1 -- concentrated/LConn1 -- A/RConn1

== system SPGF_FSK_0000_R2020b/W33 ==
  DPL : Subsystem  Commented=on  mask{N=6, Frequency=[50], R_matrix=[0.347601410823579 0.0494303286168989 0.0494305228057156 0.0494305228057156 0.0494305228057156 0.0494305228057156;0.0494303286168989 0.63357380919679 0.0494305228057156 0.0494305228057156 0.0494305228057156 0.0494305228057156;0.0494305228057156 0.0494305228057156 0.347602052073771 0.0494309698670905 0.0494311641268522 0.0494311641268522;0.0494305228057156 0.0494305228057156 0.0494309698670905 0.633574450446981 0.0494311641268522 0.0494311641268522;0.0494305228057156 0.0494305228057156 0.0494311641268522 0.0494311641268522 0.347602052073771 0.0494309698670905;0.0494305228057156 0.0494305228057156 0.0494311641268522 0.0494311641268522 0.0494309698670905 0.633574450446981], L_matrix=[0.00260859879857304 0.00242332383525137 0.00221745883616686 0.00221745883616686 0.00221745883616686 0.00221745883616686;0.00242332383525137 0.00242198857850016 0.00221745883616686 0.00221745883616686 0.00221745883616686 0.00221745883616686;0.00221745883616686 0.00221745883616686 0.00253519514382882 0.00234992018050715 0.00223977112704788 0.00223977112704788;0.00221745883616686 0.00221745883616686 0.00234992018050715 0.00234858492375594 0.00223977112704788 0.00223977112704788;0.00221745883616686 0.00221745883616686 0.00223977112704788 0.00223977112704788 0.00253519514382882 0.00234992018050715;0.00221745883616686 0.00221745883616686 0.00223977112704788 0.00223977112704788 0.00234992018050715 0.00234858492375594], C_matrix=[1.90757475136094e-07 -1.90757475136094e-07 0 0 0 0;-1.90757475136094e-07 3.66052807704686e-07 0 0 0 0;0 0 1.90757475136094e-07 -1.90757475136094e-07 0 0;0 0 -1.90757475136094e-07 3.66052807704686e-07 0 0;0 0 0 0 1.90757475136094e-07 -1.90757475136094e-07;0 0 0 0 -1.90757475136094e-07 3.66052807704686e-07], Rg_matrix=[834331.357019417 -834331.357019417 Inf Inf Inf -Inf;-834331.357019417 434786.838789375 Inf Inf Inf -Inf;Inf Inf 834331.357019417 -834331.357019417 Inf -Inf;Inf Inf -834331.357019417 434786.838789375 Inf -Inf;Inf Inf Inf Inf 834331.357019417 -834331.357019417;Inf Inf Inf Inf -834331.357019417 434786.838789375], LineLength=[0.6]}
      mask prompts: N "Number of phases [N]"; Frequency "Frequency used for rlc specification [Hz]:"; R_matrix "Resistance per unit length [Ohms/km] NxN matrix"; L_matrix "Inductance per unit length [H/km] NxN matrix"; C_matrix "Capacitance per unit length [F/km] NxN matrix"; Rg_matrix "Resistance shunt matrix 6*6 [Ohm*km]"; LineLength "Line Length(km)"
      mask init:
      | % Rloss=1/(2*pi*Frequency*C_matrix(1,1)*TangLoss);
      | Rg_matrix=Rg_matrix./LineLength;
      mask Display:
      | port_label('lconn',1,'A');
      | port_label('lconn',2,'B');
      | port_label('lconn',3,'C');
      | 
      | port_label('rconn',1,'a');
      | port_label('rconn',2,'b');
      | port_label('rconn',3,'c');
      | 
      | disp('1x95');
  Pi : Subsystem  mask{R0=0.31, X0=0.083, Cp0=0.35, tg=2, Frequency=[50], LineLength=[0.6]}
      mask prompts: R0 "Удельное активное сопротивление, Ом/км"; X0 "Удельное индуктивное сопротивление, Ом/км"; Cp0 "Удельная рабочая емкость, мкФ/км"; tg "Тангенс диэлектрических потерь, %"; Frequency "Частота сети, Гц"; LineLength "Длина линии, км"
      mask init:
      | R=R0*LineLength;
      | L=X0*LineLength/(2*pi*Frequency);
      | Cp=Cp0*LineLength*1e-6;
      | Cmf=0.1525*Cp;
      | Cfg=0.56*Cp;
      | tg_pu=tg/100;
      | 
      | Rmf=1/(Cmf*2*pi*Frequency*tg_pu);
      | Rfg=1/(Cfg*2*pi*Frequency*tg_pu);
      mask Display:
      | port_label('lconn',1,'A');
      | port_label('lconn',2,'B');
      | port_label('lconn',3,'C');
      | 
      | port_label('rconn',1,'a');
      | port_label('rconn',2,'b');
      | port_label('rconn',3,'c');
      | 
      | disp('1x95');
  Q : Subsystem
  concentrated : Subsystem  Commented=on  mask{N=6, Frequency=[50], R_matrix=[0.347601410823579 0.0494303286168989 0.0494305228057156 0.0494305228057156 0.0494305228057156 0.0494305228057156;0.0494303286168989 0.63357380919679 0.0494305228057156 0.0494305228057156 0.0494305228057156 0.0494305228057156;0.0494305228057156 0.0494305228057156 0.347602052073771 0.0494309698670905 0.0494311641268522 0.0494311641268522;0.0494305228057156 0.0494305228057156 0.0494309698670905 0.633574450446981 0.0494311641268522 0.0494311641268522;0.0494305228057156 0.0494305228057156 0.0494311641268522 0.0494311641268522 0.347602052073771 0.0494309698670905;0.0494305228057156 0.0494305228057156 0.0494311641268522 0.0494311641268522 0.0494309698670905 0.633574450446981], L_matrix=[0.00260859879857304 0.00242332383525137 0.00221745883616686 0.00221745883616686 0.00221745883616686 0.00221745883616686;0.00242332383525137 0.00242198857850016 0.00221745883616686 0.00221745883616686 0.00221745883616686 0.00221745883616686;0.00221745883616686 0.00221745883616686 0.00253519514382882 0.00234992018050715 0.00223977112704788 0.00223977112704788;0.00221745883616686 0.00221745883616686 0.00234992018050715 0.00234858492375594 0.00223977112704788 0.00223977112704788;0.00221745883616686 0.00221745883616686 0.00223977112704788 0.00223977112704788 0.00253519514382882 0.00234992018050715;0.00221745883616686 0.00221745883616686 0.00223977112704788 0.00223977112704788 0.00234992018050715 0.00234858492375594], C_matrix=[1.90757475136094e-07 -1.90757475136094e-07 0 0 0 0;-1.90757475136094e-07 3.66052807704686e-07 0 0 0 0;0 0 1.90757475136094e-07 -1.90757475136094e-07 0 0;0 0 -1.90757475136094e-07 3.66052807704686e-07 0 0;0 0 0 0 1.90757475136094e-07 -1.90757475136094e-07;0 0 0 0 -1.90757475136094e-07 3.66052807704686e-07], Rg_matrix=[834331.357019417 -834331.357019417 Inf Inf Inf -Inf;-834331.357019417 434786.838789375 Inf Inf Inf -Inf;Inf Inf 834331.357019417 -834331.357019417 Inf -Inf;Inf Inf -834331.357019417 434786.838789375 Inf -Inf;Inf Inf Inf Inf 834331.357019417 -834331.357019417;Inf Inf Inf Inf -834331.357019417 434786.838789375], LineLength=[0.6]}
      mask prompts: N "Number of phases [N]"; Frequency "Frequency [Hz]:"; R_matrix "Resistance matrix 6*6 [Ohm/km]"; L_matrix "Inductance matrix 6*6 [H/km]"; C_matrix "Capacitance matrix 6*6 [F/km]"; Rg_matrix "Resistance shunt matrix 6*6 [Ohm*km]"; LineLength "Line Length(km)"
      mask init: same as SPGF_FSK_0000_R2020b/W11/concentrated
      mask Display:
      | port_label('lconn',1,'A');
      | port_label('lconn',2,'B');
      | port_label('lconn',3,'C');
      | 
      | port_label('rconn',1,'a');
      | port_label('rconn',2,'b');
      | port_label('rconn',3,'c');
      | 
      | disp('1x95');
  a : PMIOPort  Side=Right
  b : PMIOPort  Port=2  Side=Right
  c : PMIOPort  Port=3  Side=Right
  A : PMIOPort  Port=4  Side=Left
  B : PMIOPort  Port=5  Side=Left
  C : PMIOPort  Port=6  Side=Left
  connections:
  A/RConn1 -- concentrated/LConn1 -- DPL/LConn1 -- Pi/LConn1
  C/RConn1 -- DPL/LConn3 -- concentrated/LConn3 -- Pi/LConn3
  concentrated/RConn2 -- Q/LConn2 -- DPL/RConn2 -- Pi/RConn2
  concentrated/RConn1 -- Q/LConn1 -- DPL/RConn1 -- Pi/RConn1
  concentrated/RConn3 -- Q/LConn3 -- DPL/RConn3 -- Pi/RConn3
  B/RConn1 -- concentrated/LConn2 -- DPL/LConn2 -- Pi/LConn2
  Q/RConn2 -- b/RConn1
  Q/RConn1 -- a/RConn1
  Q/RConn3 -- c/RConn1
